simulink model "verify_trajectories"  (R2021a)
settings: Solver=VariableStepAuto  StartTime=0.0  StopTime=10.0  RelTol=1e-3
settings Model: Creator=tejal  LastModifiedBy=tejal

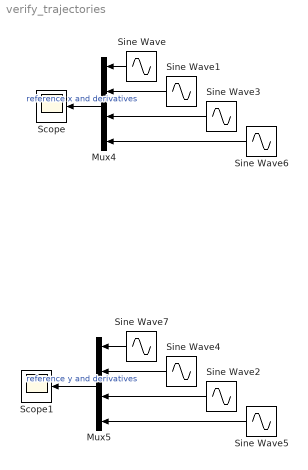
== system verify_trajectories ==
  Mux4 : Mux
  Mux5 : Mux
  Scope : Scope
  Scope1 : Scope
  Sine Wave : Sin  Amplitude=150  Phase=1.57  SampleTime=0
  Sine Wave1 : Sin  Amplitude=-150  SampleTime=0
  Sine Wave2 : Sin  Amplitude=-150  Frequency=2  SampleTime=0
  Sine Wave3 : Sin  Amplitude=-150  Phase=1.57  SampleTime=0
  Sine Wave4 : Sin  Amplitude=75  Frequency=2  Phase=1.57  SampleTime=0
  Sine Wave5 : Sin  Amplitude=-300  Frequency=2  Phase=1.57  SampleTime=0
  Sine Wave6 : Sin  Amplitude=150  SampleTime=0
  Sine Wave7 : Sin  Amplitude=37.5  Frequency=2  SampleTime=0
  wires:
  Sine Wave6/1 -> Mux4/4
  Sine Wave1/1 -> Mux4/2
  Sine Wave3/1 -> Mux4/3
  Sine Wave/1 -> Mux4/1
  Mux4/1 -> Scope/1  "reference x and derivatives"
  Sine Wave2/1 -> Mux5/3
  Sine Wave5/1 -> Mux5/4
  Sine Wave4/1 -> Mux5/2
  Sine Wave7/1 -> Mux5/1
  Mux5/1 -> Scope1/1  "reference y and derivatives"
